simulink model "qbmove_basic_example"  (R2023b)
settings: Solver=ode1  StartTime=0.0  StopTime=20  FixedStep=.002  RelTol=1e-3  EnableMultiTasking=on
libraries: qbmove_library x2, QB_pacer_lib x1, simulink x1
settings Model: Creator=laurentio  LastModifiedBy=Mattia
settings SolverCC: AlgebraicLoopSolver=TrustRegion
settings DataIOCC: LimitDataPoints=on  SaveFormat=Array  ReturnWorkspaceOutputs=off
settings OptimizationCC: LifeSpan=inf
settings DebuggingCC: UnderspecifiedInitializationDetection=Classic  MergeDetectMultiDrivingBlocksExec=none  SolverPrmCheckMsg=warning  UnconnectedInputMsg=warning  UnconnectedOutputMsg=warning  UnconnectedLineMsg=warning  AllowSymbolicDim=off  StateNameClashWarn=warning  SFUnexpectedBacktrackingDiag=warning  SFNoUnconditionalDefaultTransitionDiag=warning  SFExecutionAtInitializationDiag=none  ArithmeticOperatorsInVariantConditions=warning
settings HardwareCC: ProdBitPerPointer=32  ProdBitPerSizeT=32  ProdBitPerPtrDiffT=32  ProdLargestAtomicFloat=None  ProdIntDivRoundTo=Undefined  ProdEndianess=Unspecified  ProdWordSize=32  ProdHWDeviceType=32-bit Generic
settings ModelReferenceCC: EnableRefExpFcnMdlSchedulingChecks=on  PropagateSignalLabelsOutOfModel=off
settings SFSimCC: SimUseLocalCustomCode=off  CustomCodeUndefinedFunction=UseInterfaceOnly
settings RTWCC: RTWUseLocalCustomCode=off  DLArmComputeVersion=19.05
settings CodeAppCC: StateflowObjectComments=on
settings GRTTargetCC: TargetLangStandard=C89/C90 (ANSI)
settings ConfigComp: CovMetricSettings=dw  CovSaveCumulativeToWorkspaceVar=on  CovSaveSingleToWorkspaceVar=on  CovExternalEMLEnable=off  CovSFcnEnable=off

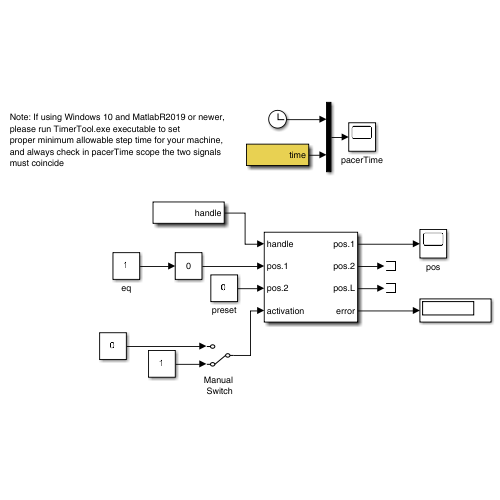
[thumbnail: Simulink's stored preview of the top-level diagram]
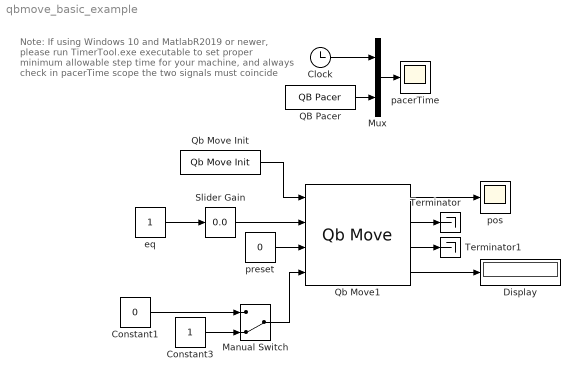
== system qbmove_basic_example ==
  note: Note: If using Windows 10 and MatlabR2019 or newer,
      | please run TimerTool.exe executable to set
      | proper minimum allowable step time for your machine,
      | and always check in pacerTime scope the two signals
      | must coincide
  Clock : Clock
  Constant1 : Constant  Value=0
  Constant3 : Constant
  Display : Display
  Manual Switch : ManualSwitch  CurrentSetting=0
  Mux : Mux  Inputs=2
  QB Pacer : QB_pacer_lib/QB Pacer  simTimePerRealTime=1
  Qb Move Init : qbmove_library/Qb Move Init  NUMBER_OF_COM='COM1'  BAUD_RATE_COM=2000000
      settings: SourceProductName=Qb Move Library
  Qb Move1 : qbmove_library/Qb Move  ID=65  ACTIVE_COMM_DIRECTIONS=Both  CONTROL_MODE=Prime Movers Positions  DAISY_CHAINING=off  MAX_ANG=0  SW_LIMIT=inf  OFFSET=0  ACTIVATE=off  WDT=0.0  UNIT=Degrees
      settings: LibrarySourceBlock=qbmove_library/qbmove  SourceProductName=Qb Move Library
  Slider Gain : simulink/Math Operations/Slider Gain  gain=0.0  low=0  high=19000
  Terminator : Terminator
  Terminator1 : Terminator
  eq : Constant
  pacerTime : Scope
  pos : Scope
  preset : Constant  Value=0
  wires:
  QB Pacer/1 -> Mux/2
  Clock/1 -> Mux/1
  Qb Move Init/1 -> Qb Move1/1
  eq/1 -> Slider Gain/1
  Constant1/1 -> Manual Switch/1
  Slider Gain/1 -> Qb Move1/2
  Constant3/1 -> Manual Switch/2
  preset/1 -> Qb Move1/3
  Qb Move1/4 -> Display/1
  Mux/1 -> pacerTime/1
  Manual Switch/1 -> Qb Move1/4
  Qb Move1/1 -> pos/1
  Qb Move1/2 -> Terminator/1
  Qb Move1/3 -> Terminator1/1
